simulink model "lucrarea3_3_sim"  (R2020b)
settings: Solver=VariableStepAuto  StartTime=0.0  StopTime=2  RelTol=1e-3
values from neighbouring files (symbols this model uses):
  J = 0.71*10^-3    (= 0.00071)    [lucrarea3_3.m]    (also in lucrarea4.m; lucrarea4_2.m; lucrarea4_3.m)
  ke = 0.33    [lucrarea3_3.m]    (also in lucrarea4.m; lucrarea4_2.m; lucrarea4_3.m)
  kEM = 0.01    [lucrarea3_3.m]    (also in lucrarea4.m; lucrarea4_2.m; lucrarea4_3.m)
  km = 0.33    [lucrarea3_3.m]    (also in lucrarea4.m; lucrarea4_2.m; lucrarea4_3.m)
  kp = 35    [lucrarea3_3.m]    (also in lucrarea4.m; lucrarea4_2.m; lucrarea4_3.m)
  La = 14.28*10^-3    (= 0.01428)    [lucrarea3_3.m]    (also in lucrarea4.m; lucrarea4_2.m; lucrarea4_3.m)
  lambda = 0.0001    [lucrarea3_2.m]    (also in lucrarea3_3.m)
  nA = 2    [lucrarea3_2.m]    (also in lucrarea3_3.m)
  nB = 1    [lucrarea3_2.m]    (also in lucrarea3_3.m)
  Orizont = 3    [lucrarea3_2.m]    (also in lucrarea3_3.m)
  P = [G1 0 0;fliplr(G2) 0;fliplr(G3)]    [lucrarea3_2.m]    (also in lucrarea3_3.m; lucrarea4_3.m = [z1; z2])
  PSI = [F1 H1;F2 H2;F3 H3]    [lucrarea3_2.m]    (also in lucrarea3_3.m)
  Q = eye(Orizont)    [lucrarea3_2.m]    (also in lucrarea3_3.m; lucrarea4.m = [1 0;0 1]; lucrarea4_2.m = [1, 0; 0, 1]; lucrarea4_3.m = [1, 0; 0, 1])
  R = zeros(N+Orizont,1);R(21:end)=1    [lucrarea3_2.m]    (also in lucrarea3_3.m; lucrarea4.m = 0.1; lucrarea4_2.m = 0.1; lucrarea4_3.m = 0.1)
  Ra = 4.2    [lucrarea3_3.m]    (also in lucrarea4.m; lucrarea4_2.m; lucrarea4_3.m)
settings Model: Creator=student  LastModifiedBy=student

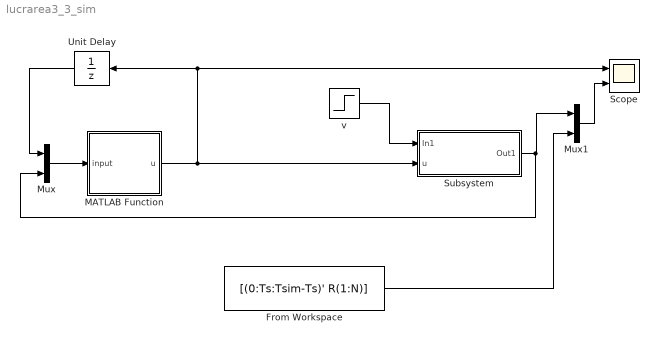
== system lucrarea3_3_sim ==
  From Workspace : FromWorkspace  VariableName=[(0:Ts:Tsim-Ts)' R(1:N)]
  MATLAB Function : MATLAB Function  TreatAsAtomicUnit=on
  Mux : Mux  Inputs=2
  Mux1 : Mux  Inputs=2
  Scope : Scope  NumInputPorts=2
  Subsystem : Subsystem
  Unit Delay : UnitDelay  SampleTime=-1  HasFrameUpgradeWarning=on
  v : Step  Time=0.6  After=-12  SampleTime=0
  wires:
  Unit Delay/1 -> Mux/1
  Mux1/1 -> Scope/2
  MATLAB Function/1(u) -> Subsystem/2(u), Scope/1, Unit Delay/1
  Mux/1 -> MATLAB Function/1(input)
  From Workspace/1 -> Mux1/2
  Subsystem/1(Out1) -> Mux/2, Mux1/1
  v/1 -> Subsystem/1(In1)

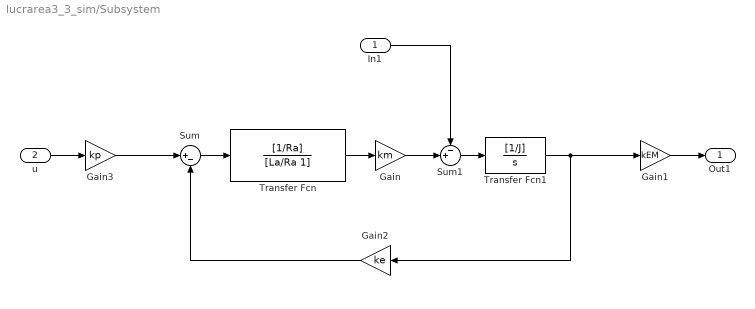
== system lucrarea3_3_sim/Subsystem ==
  In1 : Inport
  u : Inport  Port=2
  Gain : Gain  Gain=km
  Gain1 : Gain  Gain=kEM
  Gain2 : Gain  Gain=ke
  Gain3 : Gain  Gain=kp
  Sum : Sum  Inputs=|+-
  Sum1 : Sum  Inputs=-+|
  Transfer Fcn : TransferFcn  Numerator=[1/Ra]  Denominator=[La/Ra 1]
  Transfer Fcn1 : TransferFcn  Numerator=[1/J]  Denominator=[1 0]
  Out1 : Outport
  wires:
  Sum1/1 -> Transfer Fcn1/1
  Sum/1 -> Transfer Fcn/1
  Gain2/1 -> Sum/2
  Gain3/1 -> Sum/1
  Transfer Fcn/1 -> Gain/1
  Transfer Fcn1/1 -> Gain2/1, Gain1/1
  Gain/1 -> Sum1/2
  Gain1/1 -> Out1/1
  In1/1 -> Sum1/1
  u/1 -> Gain3/1

== matlab function lucrarea3_3_sim/MATLAB Function ==
  settings: updateMethod=DISCRETE
  data: input input; u output; R parameter; P parameter; PSI parameter; Q parameter; nA parameter; nB parameter; lambda parameter; Orizont parameter
% ------------------myMPC.m----------------------- %
function u = myMPC(input, R, P, PSI, Q, nA, nB, lambda, Orizont)
% to clear persistent vars in Fcn, call >>clear 'FcnName' in prompt
% clear myMPC
persistent yPast uPast k
if isempty(yPast) % initializari variabile persistente la prima rulare
yPast = zeros(2,1);
uPast = zeros(1,1);
k = 0;
end
% actualizare uPast
for i = length(uPast):-1:2
uPast(i) = uPast(i-1);
end
uPast(1) = input(1);
%%%%%%%%%%%%%%%%%%
% actualizare yPast
for i = length(yPast):-1:2
yPast(i) = yPast(i-1);
end
yPast(1) = input(2);
%%%%%%%%%%%%%%%%%%
Rs = [R(k+1) R(k+1) R(k+1)]';
% eyeO=[1 0 0;0 1 0;0 0 1];
Sol = -inv(P'*Q*P + lambda*eye(3)) * P' * Q * (PSI*[yPast;uPast]-Rs);
u = Sol(1);
k = k+1; %salt la pasul urmator
end % end myMPC
%-----------------------------------------------------------%
